simulink subsystem "AnalogAcquisition"  (R2023b)
settings: Solver=VariableStepAuto  StartTime=0.0  StopTime=10.0  RelTol=1e-3
undefined symbols (not defined in the file): ADC_CountMax, ADC_VMax
libraries: c2802xlib x1
settings Model: Creator=rodri  LastModifiedBy=rodri

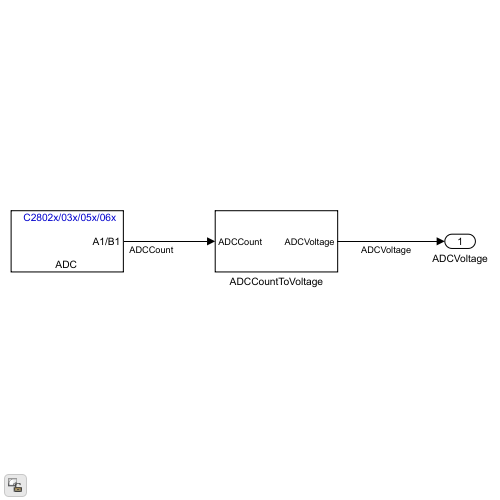
[thumbnail: Simulink's stored preview of the top-level diagram]
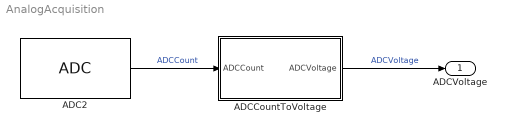
== system AnalogAcquisition ==
  ADC2 : c2802xlib/ADC  blkParamProc=C2000  ADCModule=1  samplingMode=Simultaneous sample mode  ADCResolution=12-bit (Single-ended input)  useSOC1=SOC0  useSOC2=SOC0_SOC1  SOCAcquisitionWindow=7  SOCTriggerSource=ePWM1_ADCSOCA  SOCInterruptTrigger=No ADCINT  Ts=0.001  dType=single  postInterrupt=on  interruptSel=ADCINT1  ADCINTContinuous=on  endma=off  chdma=1  conv1=ADCINA0  conv2=ADCINA1 and ADCINB1  conv1_Type4=ADCIN0  conv2_Type4=ADCIN0 and ADCIN1
  ADCCountToVoltage : Subsystem
  ADCVoltage : Outport
  wires:
  ADC2/1 -> ADCCountToVoltage/1(ADCCount)  "ADCCount"
  ADCCountToVoltage/1(ADCVoltage) -> ADCVoltage/1  "ADCVoltage"

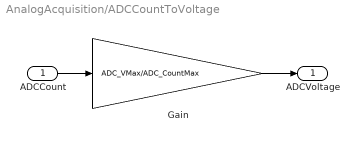
== system AnalogAcquisition/ADCCountToVoltage ==
  ADCCount : Inport
  Gain : Gain  Gain=ADC_VMax/ADC_CountMax
  ADCVoltage : Outport
  wires:
  Gain/1 -> ADCVoltage/1
  ADCCount/1 -> Gain/1
